simulink model "dsvf"  (Simulink 7.1)
settings: Solver=FixedStepDiscrete  StartTime=0.0  StopTime=1  FixedStep=sampleTime  RelTol=1e-3
values from neighbouring files (symbols this model uses):
  period = 11    [dsvf_demo.m]    (also in lamps_demo.m = 140; onehoist_demo.m = 208; simple_init.m = w/data.frequency)
  sampleTime = 1/220000    (= 4.54545454545e-06)    [dsvf_demo.m]
  TS = alg1rjcmax(T,p)    [alg1rjcmax_demo.m]    (also in alg1sumuj_demo.m = alg1sumuj(T,p); alg1sumwjdj_demo.m = alg1sumwjdj(T, prob); brucker76_demo.m = brucker76(T,prob,4); coffmangraham_demo.m = coffmangraham(T,p))
settings Model: Creator=capekr1  LastModifiedBy=Roman
settings DebuggingCC: SaveWithParameterizedLinksMsg=none  SignalResolutionControl=TryResolveAllWithWarning  MultiTaskDSMMsg=warning  MultiTaskCondExecSysMsg=none
settings RTWCC: IncludeERTFirstTime=on
settings GRTTargetCC: TargetFcnLib=ansi_tfl_tmw.mat

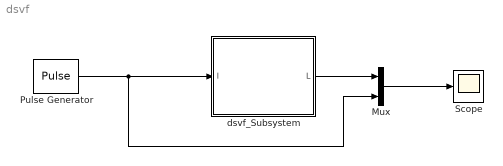
== system dsvf ==
  Mux : Mux  Inputs=2
  Pulse Generator : DiscretePulseGenerator  PulseType=Time based  Period=1/10  PulseWidth=50
  Scope : Scope
      settings: TimeRange=1  YMin=-0.5  YMax=1.5
  dsvf_Subsystem : Subsystem
  wires:
  Pulse Generator/1 -> dsvf_Subsystem/1(I), Mux/2
  dsvf_Subsystem/1(L) -> Mux/1
  Mux/1 -> Scope/1

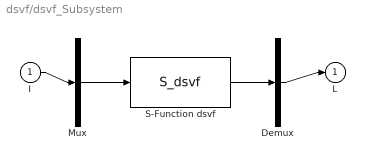
== system dsvf/dsvf_Subsystem ==
  I : Inport
  Demux : Demux  Outputs=1
  Mux : Mux  Inputs=1
  S-Function dsvf : S-Function  FunctionName=S_dsvf  Parameters=sampleTime,TS,period  EnableBusSupport=off
  L : Outport
  wires:
  Mux/1 -> S-Function dsvf/1
  S-Function dsvf/1 -> Demux/1
  I/1 -> Mux/1
  Demux/1 -> L/1
